simulink model "BouncingBoxLooping"  (R2014b)
settings: Solver=ode45  StartTime=0.0  StopTime=100.0  RelTol=1e-3
libraries: vrlib x2
settings Model: Creator=Ben  LastModifiedBy=Ben

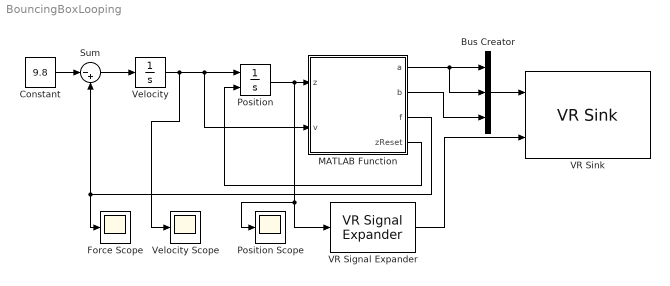
== system BouncingBoxLooping ==
  Bus Creator : BusCreator  Inputs=3
  Constant : Constant  Value=9.8
  Force Scope : Scope
      settings: TimeRange=100  YMin=0  YMax=400
  MATLAB Function : MATLAB Function  TreatAsAtomicUnit=on
  Position : Integrator  ExternalReset=rising  InitialCondition=20
  Position Scope : Scope
      settings: YMin=0  YMax=20
  Sum : Sum  Inputs=|-+
  VR Signal Expander : vrlib/VR Signal Expander  outwidth=3  outidx=[3]
  VR Sink : vrlib/VR Sink  InstantiateOnLoad=on  SampleTime=0.1  ViewEnable=on  RemoteChange=off  RemoteView=on  FieldsWritten=BoxTransform.scale.3.1.1.double#BoxTransform.translation.3.1.1.double  WorldFileName=BouncingBoxSimulink.wrl  WorldDescription=VRML scene BouncingBoxSimulink.wrl  AutoView=off  VideoDimensions=[]  AllowVariableSize=off
  Velocity : Integrator
  Velocity Scope : Scope
      settings: YMin=-20  YMax=20  SaveName=ScopeData2
  wires:
  MATLAB Function/3(f) -> Sum/2, Force Scope/1
  Constant/1 -> Sum/1
  Sum/1 -> Velocity/1
  VR Signal Expander/1 -> VR Sink/2
  MATLAB Function/1(a) -> Bus Creator/2, Bus Creator/1
  Bus Creator/1 -> VR Sink/1
  MATLAB Function/2(b) -> Bus Creator/3
  MATLAB Function/4(zReset) -> Position/2
  Position/1 -> Position Scope/1, VR Signal Expander/1, MATLAB Function/1(z)
  Velocity/1 -> MATLAB Function/2(v), Position/1, Velocity Scope/1

== matlab function BouncingBoxLooping/MATLAB Function ==
  data: a output; b output; z input; f output; v input; zReset output
% First edition date: Oct/10/2014
% Matlab 2014b Simulink VRtool
% Referance:http://www.mathworks.com/help/sl3d/examples/bouncing-ball.html"
% Revised date: Oct/17/2014
% 

function [a, b,f, zReset] = fcn(z, v)
%#codegen
f2=0;
zReset=0;   % Z position Reset signal =0 --> No reset

% Do not let z goes to negtive
if z<1e-4
    z=1e-4;
end

if z<1.5  % during compression
    f1=600*(1.5-z); % spring compression equations
    if v<0 % decelerate the ball
        f2=-6*v;
% when the deceleration force dies out, zReset=1 trigers z back to initial value.
        if abs(f2)<.7  
            zReset=1;   
        end
    end
    a=sqrt(1.5^3/z);
    b=z;
else      % during free fall
    f1=0;
    a=1.5;
    b=1.5;    
end 
f=f1+f2; % accumulated force
